simulink model "Model2"  (R2013b)
settings: Solver=ode45  StartTime=0.0  StopTime=20.0  MaxStep=1e-5  MinStep=1e-6  RelTol=1e-3
undefined symbols (not defined in the file or in its folder): i
settings Model: Creator=user  LastModifiedBy=user
settings SolverCC: InitialStep=1e-6

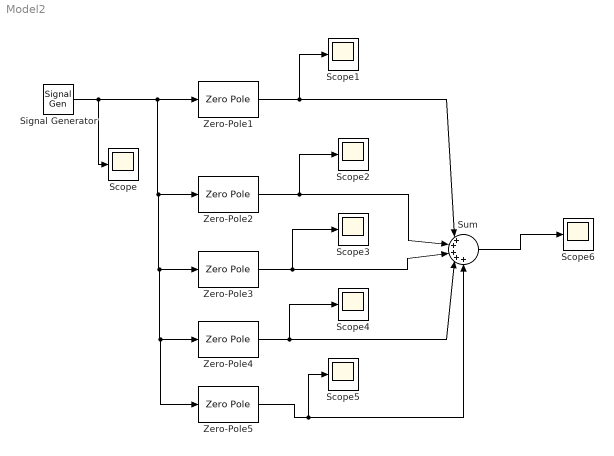
== system Model2 ==
  Scope{,1..6} (7 alike) : Scope
      Scope settings: TickLabels=on  TimeRange=1  YMin=-1  YMax=1
      Scope1 settings: TickLabels=on  TimeRange=1
      Scope2 settings: TickLabels=on  TimeRange=1  YMin=-0.0125  YMax=0.0125  SaveName=ScopeData2
      Scope3 settings: TickLabels=on  TimeRange=1  YMin=-0.5  YMax=0.5  SaveName=ScopeData3
      Scope4 settings: TickLabels=on  TimeRange=1  YMin=-0.0125  YMax=0.0125  SaveName=ScopeData4
      Scope5 settings: TickLabels=on  TimeRange=1  YMin=-0.3  YMax=0.3  SaveName=ScopeData5
      Scope6 settings: TickLabels=on  TimeRange=1  YMin=-1.25  YMax=1.25  SaveName=ScopeData6
  Signal Generator : SignalGenerator  WaveForm=square  Frequency=25
  Sum : Sum  Inputs=|+++++
  Zero-Pole1 : ZeroPole  Zeros=[0]  Poles=[-1*2*pi*25*0.005+i*1*2*pi*25*0.9999875, -1*2*pi*25*0.005-i*1*2*pi*25*0.9999875]  Gain=[1*2*pi*25*0.01]
  Zero-Pole2 : ZeroPole  Zeros=[0]  Poles=[-2*2*pi*25*0.005+i*2*2*pi*25*0.9999875, -2*2*pi*25*0.005-i*2*2*pi*25*0.9999875]  Gain=[2*2*pi*25*0.01]
  Zero-Pole3 : ZeroPole  Zeros=[0]  Poles=[-3*2*pi*25*0.005+i*3*2*pi*25*0.9999875, -3*2*pi*25*0.005-i*3*2*pi*25*0.9999875]  Gain=[3*2*pi*25*0.01]
  Zero-Pole4 : ZeroPole  Zeros=[0]  Poles=[-4*2*pi*25*0.005+i*4*2*pi*25*0.9999875, -4*2*pi*25*0.005-i*4*2*pi*25*0.9999875]  Gain=[4*2*pi*25*0.01]
  Zero-Pole5 : ZeroPole  Zeros=[0]  Poles=[-5*2*pi*25*0.005+i*5*2*pi*25*0.9999875, -5*2*pi*25*0.005-i*5*2*pi*25*0.9999875]  Gain=[5*2*pi*25*0.01]
  wires:
  Zero-Pole1/1 -> Scope1/1, Sum/1
  Signal Generator/1 -> Scope/1, Zero-Pole5/1, Zero-Pole4/1, Zero-Pole3/1, Zero-Pole2/1, Zero-Pole1/1
  Zero-Pole2/1 -> Scope2/1, Sum/2
  Zero-Pole3/1 -> Scope3/1, Sum/3
  Zero-Pole4/1 -> Scope4/1, Sum/4
  Zero-Pole5/1 -> Scope5/1, Sum/5
  Sum/1 -> Scope6/1
